simulink model "transmit_LSF"  (R2024b)
settings: Solver=FixedStepAuto  StartTime=0.0  StopTime=0  FixedStep=1  RelTol=1e-3
values from neighbouring files (symbols this model uses):
  SBLSF = hexToArray(SBLSF,1)    [Full_transmit.m]
settings Model: Creator=fredr  LastModifiedBy=SERGIO

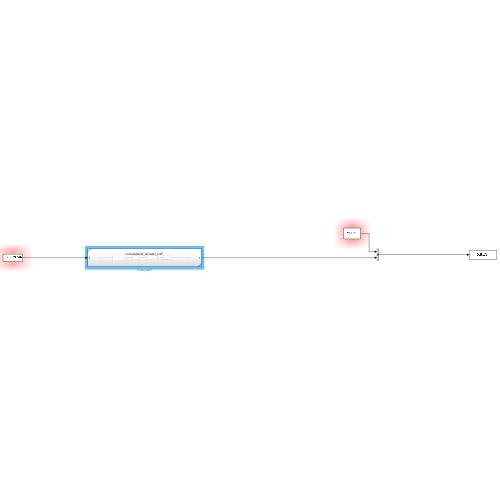
[thumbnail: Simulink's stored preview of the top-level diagram]
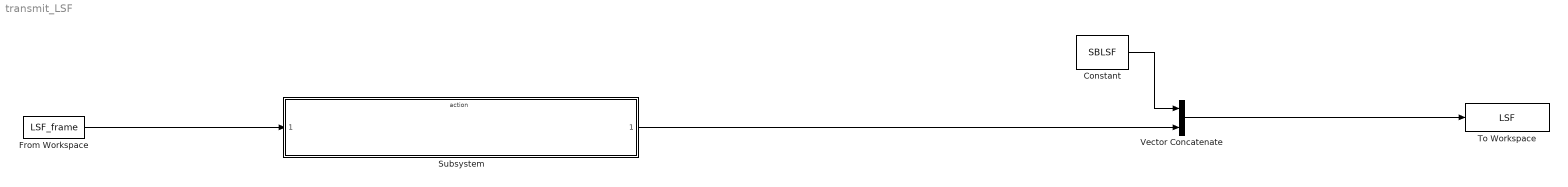
== system transmit_LSF ==
  Constant : Constant  Value=SBLSF
  From Workspace : FromWorkspace  VariableName=LSF_frame
  Subsystem : Subsystem  ReferencedSubsystem=convolutional_encoder_LSF
  To Workspace : ToWorkspace  VariableName=LSF  SampleTime=-1
      settings: Save2DSignal=2-D array (concatenate along first dimension)
  Vector Concatenate : Concatenate
  wires:
  Vector Concatenate/1 -> To Workspace/1
  Constant/1 -> Vector Concatenate/1
  From Workspace/1 -> Subsystem/1
  Subsystem/1 -> Vector Concatenate/2
